simulink library "HvsOpen"  (Simulink 7.8)
settings: Solver=ode45  StartTime=0.0  StopTime=10.0  RelTol=1e-3
(part 2 of 2)

== system HvsOpen/DATAPACK/dec2byte8/Subsystem7 ==
  In1 : Inport
  Constant8 : Constant  Value=power
  Constant9 : Constant  Value=2
  Math Function : Math  Operator=pow  SaturateOnIntegerOverflow=on
  Product : Product  RndMeth=Zero
  Out1 : Outport
  wires:
  Product/1 -> Out1/1
  In1/1 -> Product/1
  Math Function/1 -> Product/2
  Constant9/1 -> Math Function/1
  Constant8/1 -> Math Function/2

== system HvsOpen/DATAPACK/dec2byte9/Subsystem ==
  In1 : Inport
  Constant8 : Constant  Value=power
  Constant9 : Constant  Value=2
  Math Function : Math  Operator=pow  SaturateOnIntegerOverflow=on
  Product : Product  RndMeth=Zero
  Out1 : Outport
  wires:
  Product/1 -> Out1/1
  In1/1 -> Product/1
  Math Function/1 -> Product/2
  Constant9/1 -> Math Function/1
  Constant8/1 -> Math Function/2

== system HvsOpen/DATAPACK/dec2byte9/Subsystem1 ==
  In1 : Inport
  Constant8 : Constant  Value=power
  Constant9 : Constant  Value=2
  Math Function : Math  Operator=pow  SaturateOnIntegerOverflow=on
  Product : Product  RndMeth=Zero
  Out1 : Outport
  wires:
  Constant8/1 -> Math Function/2
  Constant9/1 -> Math Function/1
  Math Function/1 -> Product/2
  In1/1 -> Product/1
  Product/1 -> Out1/1

== system HvsOpen/DATAPACK/dec2byte9/Subsystem2 ==
  In1 : Inport
  Constant8 : Constant  Value=power
  Constant9 : Constant  Value=2
  Math Function : Math  Operator=pow  SaturateOnIntegerOverflow=on
  Product : Product  RndMeth=Zero
  Out1 : Outport
  wires:
  Product/1 -> Out1/1
  In1/1 -> Product/1
  Math Function/1 -> Product/2
  Constant9/1 -> Math Function/1
  Constant8/1 -> Math Function/2

== system HvsOpen/DATAPACK/dec2byte9/Subsystem3 ==
  In1 : Inport
  Constant8 : Constant  Value=power
  Constant9 : Constant  Value=2
  Math Function : Math  Operator=pow  SaturateOnIntegerOverflow=on
  Product : Product  RndMeth=Zero
  Out1 : Outport
  wires:
  Constant8/1 -> Math Function/2
  Constant9/1 -> Math Function/1
  Math Function/1 -> Product/2
  In1/1 -> Product/1
  Product/1 -> Out1/1

== system HvsOpen/DATAPACK/dec2byte9/Subsystem4 ==
  In1 : Inport
  Constant8 : Constant  Value=power
  Constant9 : Constant  Value=2
  Math Function : Math  Operator=pow  SaturateOnIntegerOverflow=on
  Product : Product  RndMeth=Zero
  Out1 : Outport
  wires:
  Product/1 -> Out1/1
  In1/1 -> Product/1
  Math Function/1 -> Product/2
  Constant9/1 -> Math Function/1
  Constant8/1 -> Math Function/2

== system HvsOpen/DATAPACK/dec2byte9/Subsystem5 ==
  In1 : Inport
  Constant8 : Constant  Value=power
  Constant9 : Constant  Value=2
  Math Function : Math  Operator=pow  SaturateOnIntegerOverflow=on
  Product : Product  RndMeth=Zero
  Out1 : Outport
  wires:
  Constant8/1 -> Math Function/2
  Constant9/1 -> Math Function/1
  Math Function/1 -> Product/2
  In1/1 -> Product/1
  Product/1 -> Out1/1

== system HvsOpen/DATAPACK/dec2byte9/Subsystem6 ==
  In1 : Inport
  Constant8 : Constant  Value=power
  Constant9 : Constant  Value=2
  Math Function : Math  Operator=pow  SaturateOnIntegerOverflow=on
  Product : Product  RndMeth=Zero
  Out1 : Outport
  wires:
  Product/1 -> Out1/1
  In1/1 -> Product/1
  Math Function/1 -> Product/2
  Constant9/1 -> Math Function/1
  Constant8/1 -> Math Function/2

== system HvsOpen/DATAPACK/dec2byte9/Subsystem7 ==
  In1 : Inport
  Constant8 : Constant  Value=power
  Constant9 : Constant  Value=2
  Math Function : Math  Operator=pow  SaturateOnIntegerOverflow=on
  Product : Product  RndMeth=Zero
  Out1 : Outport
  wires:
  Constant8/1 -> Math Function/2
  Constant9/1 -> Math Function/1
  Math Function/1 -> Product/2
  In1/1 -> Product/1
  Product/1 -> Out1/1
